simulink model "saccade_lin"  (Simulink 7.4)
settings: Solver=ode45  SolverMode=SingleTasking  StartTime=0.0  StopTime=0.4  RelTol=1e-5  AbsTol=1e-8
settings Model: Creator=johnvo  LastModifiedBy=johnvo
settings DataIOCC: LimitDataPoints=off
settings OptimizationCC: BlockReduction=off  BooleanDataType=off
settings DebuggingCC: SaveWithParameterizedLinksMsg=none  SignalResolutionControl=TryResolveAllWithWarning  SolverPrmCheckMsg=none  MultiTaskDSMMsg=warning  MultiTaskCondExecSysMsg=none  StrictBusMsg=None
settings HardwareCC: TargetUnknown=on
settings RTWCC: IncludeERTFirstTime=on

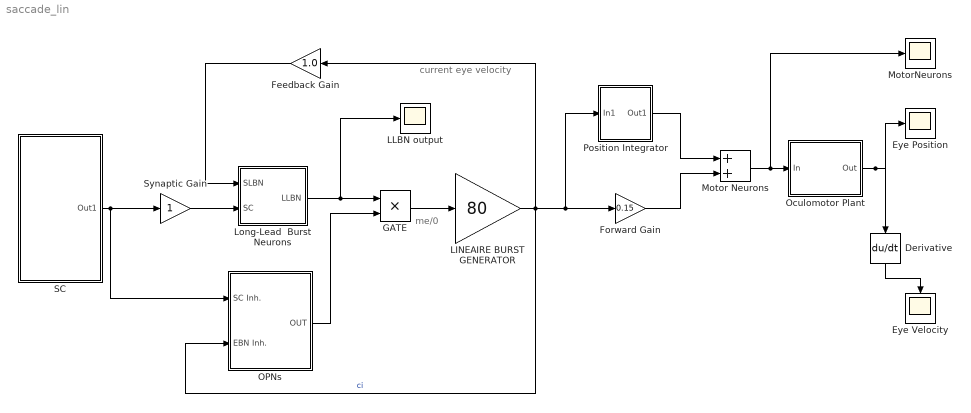
== system saccade_lin ==
  note: current eye velocity
  note: me/0
  Derivative : Derivative
  Eye Position : Scope
      settings: TickLabels=on  YMin=-10  YMax=50  DataFormat=Array
  Eye Velocity : Scope
      settings: TickLabels=on  YMin=-50  YMax=700  DataFormat=Array
  "Feedback Gain " : Gain  Gain=1.0  SaturateOnIntegerOverflow=on  OutDataTypeStr=Inherit: Same as input  ParamDataTypeStr=Inherit: Same as input
  Forward Gain : Gain  Gain=0.15  SaturateOnIntegerOverflow=on  OutDataTypeStr=Inherit: Same as input  ParamDataTypeStr=Inherit: Same as input
  GATE : Product  SaturateOnIntegerOverflow=on  RndMeth=Zero  InputSameDT=on  OutDataTypeStr=Inherit: Same as first input
  LINEAIRE BURST GENERATOR : Gain  Description=BRST  Gain=80  ParameterDataType=fixdt(1, 16)  ParameterScaling=2^0  OutDataType=fixdt(1, 16)  OutScaling=2^0
  LLBN output : Scope
      settings: TickLabels=on  YMax=20  DataFormat=Array
  Long-Lead  Burst Neurons : Subsystem
      mask Type: Long-Lead Burst Neurons
      mask Description: Comparator that integrates the difference between a desired eye velocity signal  from the Superior Colliculus, and the current eye velocity from the Short-Lead Burst Neurons.
      mask Display:
      | text(0.5,0.5,'LLBN')
      | text(0.05,0.8,'- slbn')
      | text(0.05,0.2,'+ SC')
  Motor Neurons : Sum  SaturateOnIntegerOverflow=on  InputSameDT=on  OutDataTypeStr=Inherit: Same as first input
  MotorNeurons : Scope
      settings: TickLabels=on  YMin=-10  YMax=150  DataFormat=Array
  "OPNs " : Subsystem  mask(OPNs){DEL=15, G=0.2, bias=80}
      mask prompts: DEL "Trigger Delay (ms)"; G "SC Gain"; bias "BIAS  (Hz)"
      mask help:
      | Pause system that triggers eye by an attenuated SC input burst, and inhibits the burst generator during fixations with intensity Bias.
      | During the saccade, the burst generator inhibits the pause cells.
      mask Help:
      | User controls:
      |         Bias level (in Hz)   (defines the Pause neuron activity level during fixation)
      |         SC burst, of which the Gain can be set.
      |          Trigger delay (in ms), which determines saccade onset (and kinematics!)
      | Inputs:
      |         SC burst, attenuated by OPN inhibition gain, and delayed.
      |         Horizontal eye velocity (5ms latch delay)
      | Outputs:
      |          either 0 or 1
      mask Display:
      | plot([.1 .3],[.4 .4])
      | plot([.3 .5],[.4 .6])
      | plot([.5 .65],[.4 .4])
      | text(.65,.65,'0')
      | text(.57,.40,'me')
      | 
      | plot([.1 .7],[.3 .3])  plot([.1 .1],[.3 .7])
      | plot([.1 .7],[.7 .7])  plot([.7 .7],[.3 .7])
  Oculomotor Plant : Subsystem  mask(Oculomotor Plant){T1=0.15, T2=0.020}
      mask prompts: T1 "High Time Constant (T1)"; T2 "Low Time Constant (T2)"
      mask help:
      | Second order model of the oculomotor plant
      | as proposed by Robinson and colleagues.
      |
      |  Model equation in Laplace notation:
      |
      |                         1
      |  H(s) = ---------------
      |             (1 + s.T1) . (1 + s.T2)
      mask Help:
      | T1 is the `high' time constant (muscle twitch relaxation time)
      |       default value: 0.15 sec
      |  T2 is the `low' time constant (muscle twitch contraction time)
      |       default value: 0.012 sec
      mask Display:
      | plot([0 0.1 0.15 0.2 0.25 0.3 0.5 0.7 0.9 1], [0 0.1 0.4 0.65 0.66 0.55 0.35 0.15 0.05 0])
      | text(0.04,0.5,'T2') text(0.55,0.5, 'T1')
  Position Integrator : Subsystem  mask(Eye Position Integrator){G=1.0}
      mask prompts: G "Integrator Gain"
      mask Display: text(.35,.5,'INT')
  "SC " : Subsystem  mask{FR=800, D=50}
      mask prompts: FR "Firing Rate (FR, in Hz)"; D "Burst Duration (D,  in msec)"
      mask help: The Superior Colliculus issues a burst of spikes of height FR (Hz) and duration D (in sec).
      mask Display:
      | text(.2,.85,'SC BURST')
      | plot([.2 .35,.36,.65,.66,.8],[.05,.05,.5,.5,.05,.05])
      | text(.15,.5,'FR')
      | text(.5,.05,'D')
  Synaptic Gain : Gain  SaturateOnIntegerOverflow=on  OutDataTypeStr=Inherit: Same as input  ParamDataTypeStr=Inherit: Same as input
  wires:
  "SC "/1(Out1) -> "OPNs "/1(SC Inh.), Synaptic Gain/1
  Derivative/1 -> Eye Velocity/1
  Oculomotor Plant/1(Out) -> Derivative/1, Eye Position/1
  Long-Lead  Burst Neurons/1(LLBN) -> LLBN output/1, GATE/1
  GATE/1 -> LINEAIRE BURST GENERATOR/1
  "Feedback Gain "/1 -> Long-Lead  Burst Neurons/1(SLBN)
  "OPNs "/1(OUT) -> GATE/2
  Synaptic Gain/1 -> Long-Lead  Burst Neurons/2(SC)
  Position Integrator/1(Out1) -> Motor Neurons/1
  Forward Gain/1 -> Motor Neurons/2
  Motor Neurons/1 -> MotorNeurons/1, Oculomotor Plant/1("In ")
  LINEAIRE BURST GENERATOR/1 -> "Feedback Gain "/1, "OPNs "/2(EBN Inh.), Position Integrator/1(In1), Forward Gain/1  "ci"

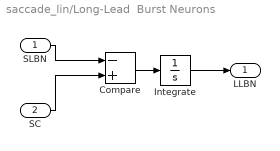
== system saccade_lin/Long-Lead  Burst Neurons ==
  SLBN : Inport
  SC : Inport  Port=2
  "Compare " : Sum  Inputs=-+  SaturateOnIntegerOverflow=on  InputSameDT=on  OutDataTypeStr=Inherit: Same as first input
  Integrate : Integrator
  LLBN : Outport  InitialOutput=0
  wires:
  SC/1 -> "Compare "/2
  Integrate/1 -> LLBN/1
  SLBN/1 -> "Compare "/1
  "Compare "/1 -> Integrate/1

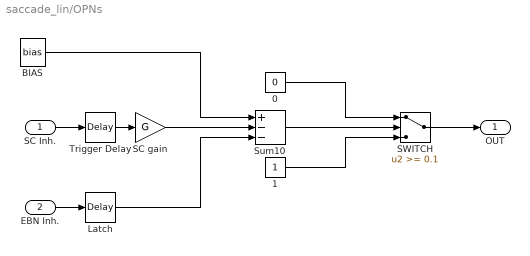
== system saccade_lin/OPNs  ==
  SC Inh. : Inport
  EBN Inh. : Inport  Port=2
  0 : Constant  Value=0
  1 : Constant
  BIAS : Constant  Value=bias
  Latch : TransportDelay  DelayTime=0.005
  SC gain : Gain  Gain=G  SaturateOnIntegerOverflow=on  OutDataTypeStr=Inherit: Same as input  ParamDataTypeStr=Inherit: Same as input
  SWITCH : Switch  Threshold=0.1  SaturateOnIntegerOverflow=on  InputSameDT=on
  Sum10 : Sum  Inputs=+--  SaturateOnIntegerOverflow=on  InputSameDT=on  OutDataTypeStr=Inherit: Same as first input
  Trigger Delay : TransportDelay  DelayTime=0.001*DEL
  OUT : Outport  InitialOutput=0
  wires:
  EBN Inh./1 -> Latch/1
  Latch/1 -> Sum10/3
  Trigger Delay/1 -> SC gain/1
  SC Inh./1 -> Trigger Delay/1
  SC gain/1 -> Sum10/2
  Sum10/1 -> SWITCH/2
  1/1 -> SWITCH/3
  0/1 -> SWITCH/1
  SWITCH/1 -> OUT/1
  BIAS/1 -> Sum10/1

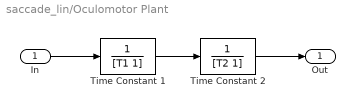
== system saccade_lin/Oculomotor Plant ==
  "In " : Inport
  Time Constant 1 : TransferFcn  Denominator=[T1 1]
  Time Constant 2 : TransferFcn  Denominator=[T2 1]
  Out : Outport  InitialOutput=0
  wires:
  Time Constant 2/1 -> Out/1
  "In "/1 -> Time Constant 1/1
  Time Constant 1/1 -> Time Constant 2/1

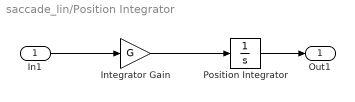
== system saccade_lin/Position Integrator ==
  In1 : Inport
  Integrator Gain : Gain  Gain=G  SaturateOnIntegerOverflow=on  OutDataTypeStr=Inherit: Same as input  ParamDataTypeStr=Inherit: Same as input
  Position Integrator : Integrator
  Out1 : Outport  InitialOutput=0
  wires:
  Integrator Gain/1 -> Position Integrator/1
  Position Integrator/1 -> Out1/1
  In1/1 -> Integrator Gain/1

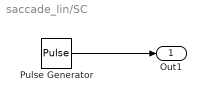
== system saccade_lin/SC  ==
  Pulse Generator : DiscretePulseGenerator  PulseType=Time based  Amplitude=FR  Period=1  PulseWidth=D * 0.1  PhaseDelay=0.05  SampleTime=1
  Out1 : Outport  InitialOutput=0
  wires:
  Pulse Generator/1 -> Out1/1
